simulink model "farmokinetic"  (R2015b)
settings: Solver=ode45  StartTime=0.0  StopTime=100  MaxStep=0.001  RelTol=1e-6
undefined symbols (not defined in the file): e, k1, k12, k21, kel, M, Time
libraries: dspswit3 x2
settings Model: Creator=DNikolaev  LastModifiedBy=DNikolaev

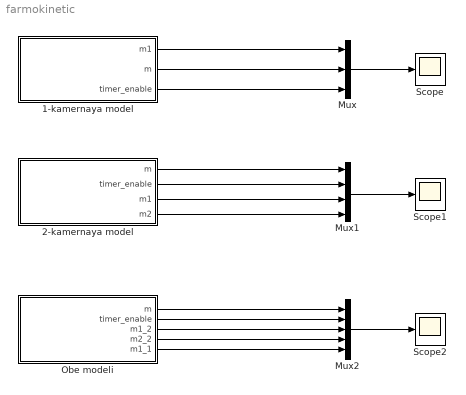
== system farmokinetic ==
  1-kamernaya model : Subsystem
  2-kamernaya model : Subsystem
  Mux : Mux  Inputs=3
  Mux1 : Mux
  Mux2 : Mux  Inputs=5
  Obe modeli : Subsystem
  Scope : Scope
  Scope1 : Scope
  Scope2 : Scope
  wires:
  1-kamernaya model/2(m) -> Mux/2
  1-kamernaya model/1(m1) -> Mux/1
  1-kamernaya model/3(timer_enable) -> Mux/3
  Mux/1 -> Scope/1
  2-kamernaya model/1(m) -> Mux1/1
  2-kamernaya model/2(timer_enable) -> Mux1/2
  Mux1/1 -> Scope1/1
  2-kamernaya model/3(m1) -> Mux1/3
  2-kamernaya model/4(m2) -> Mux1/4
  Mux2/1 -> Scope2/1
  Obe modeli/1(m) -> Mux2/1
  Obe modeli/2(timer_enable) -> Mux2/2
  Obe modeli/3(m1_2) -> Mux2/3
  Obe modeli/4(m2_2) -> Mux2/4
  Obe modeli/5(m1_1) -> Mux2/5

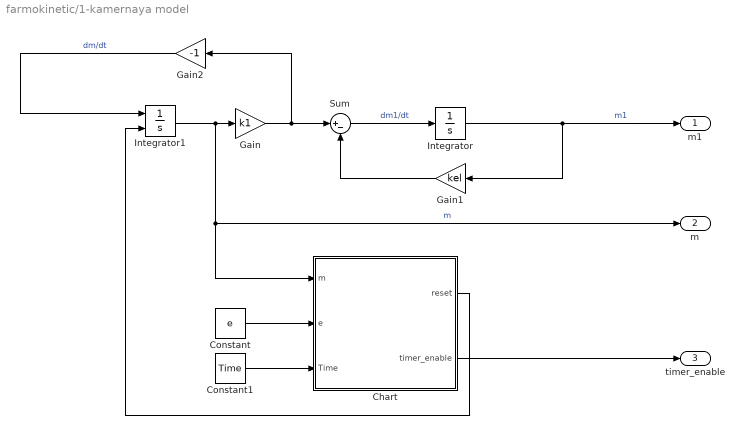
== system farmokinetic/1-kamernaya model ==
  Chart : Stateflow chart  TreatAsAtomicUnit=on
  Constant : Constant  Value=e
  Constant1 : Constant  Value=Time
  Gain : Gain  Gain=k1
  Gain1 : Gain  Gain=kel
  Gain2 : Gain  Gain=-1
  Integrator : Integrator
  Integrator1 : Integrator  ExternalReset=rising  InitialCondition=M
  Sum : Sum  Inputs=|+-
  m1 : Outport
  m : Outport  Port=2
  timer_enable : Outport  Port=3
  wires:
  Integrator/1 -> m1/1, Gain1/1  "m1"
  Sum/1 -> Integrator/1  "dm1/dt"
  Integrator1/1 -> Chart/1(m), m/1, Gain/1  "m"
  Gain/1 -> Gain2/1, Sum/1
  Gain1/1 -> Sum/2
  Gain2/1 -> Integrator1/1  "dm/dt"
  Chart/1(reset) -> Integrator1/2
  Chart/2(timer_enable) -> timer_enable/1
  Constant/1 -> Chart/2(e)
  Constant1/1 -> Chart/3(Time)

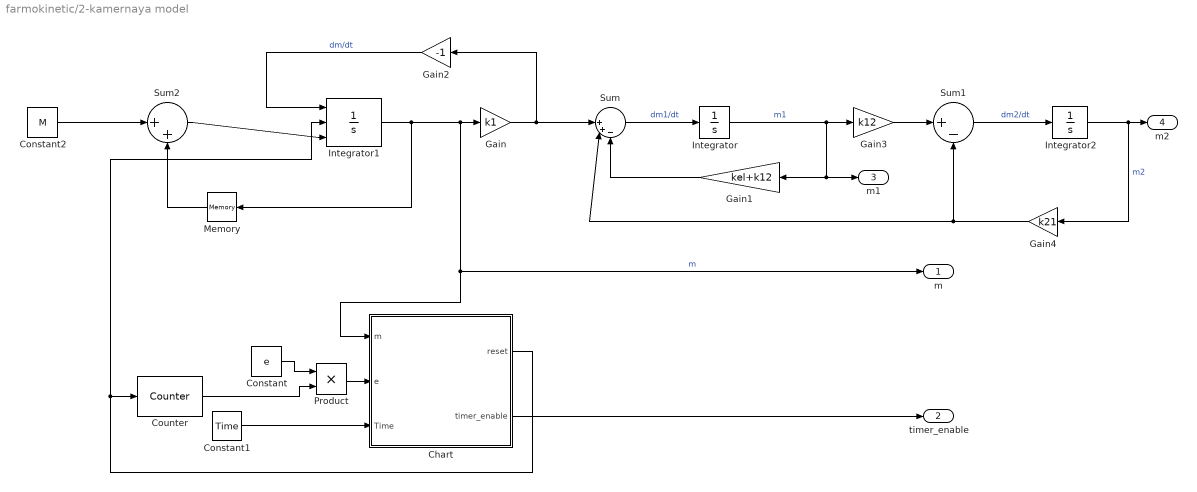
== system farmokinetic/2-kamernaya model ==
  Chart : Stateflow chart  TreatAsAtomicUnit=on
  Constant : Constant  Value=e
  Constant1 : Constant  Value=Time
  Constant2 : Constant  Value=M
  Counter : dspswit3/Counter  Direction=Up  CountEvent=Rising edge  CounterSize=User defined  MaxCount=50000  InitialCount=1  Output=Count  HitValue=32  ResetInput=off  SamplesPerFrame=1  Ts=1  CntDtype=double  HitDtype=Logical
  Gain : Gain  Gain=k1
  Gain1 : Gain  Gain=kel+k12
  Gain2 : Gain  Gain=-1
  Gain3 : Gain  Gain=k12
  Gain4 : Gain  Gain=k21
  Integrator : Integrator
  Integrator1 : Integrator  ExternalReset=rising  InitialConditionSource=external  InitialCondition=M
  Integrator2 : Integrator
  Memory : Memory
  Product : Product
  Sum : Sum  Inputs=||++-
  Sum1 : Sum  Inputs=|+-
  Sum2 : Sum  Inputs=|++
  m : Outport
  timer_enable : Outport  Port=2
  m1 : Outport  Port=3
  m2 : Outport  Port=4
  wires:
  Gain2/1 -> Integrator1/1  "dm/dt"
  Integrator1/1 -> Memory/1, Chart/1(m), m/1, Gain/1  "m"
  Gain1/1 -> Sum/3
  Gain/1 -> Sum/1, Gain2/1
  Sum/1 -> Integrator/1  "dm1/dt"
  Integrator/1 -> Gain1/1, m1/1, Gain3/1  "m1"
  Gain3/1 -> Sum1/1
  Integrator2/1 -> Gain4/1, m2/1  "m2"
  Gain4/1 -> Sum1/2, Sum/2
  Sum1/1 -> Integrator2/1  "dm2/dt"
  Constant2/1 -> Sum2/1
  Sum2/1 -> Integrator1/3
  Memory/1 -> Sum2/2
  Chart/1(reset) -> Integrator1/2, Counter/1
  Chart/2(timer_enable) -> timer_enable/1
  Constant/1 -> Product/1
  Constant1/1 -> Chart/3(Time)
  Product/1 -> Chart/2(e)
  Counter/1 -> Product/2

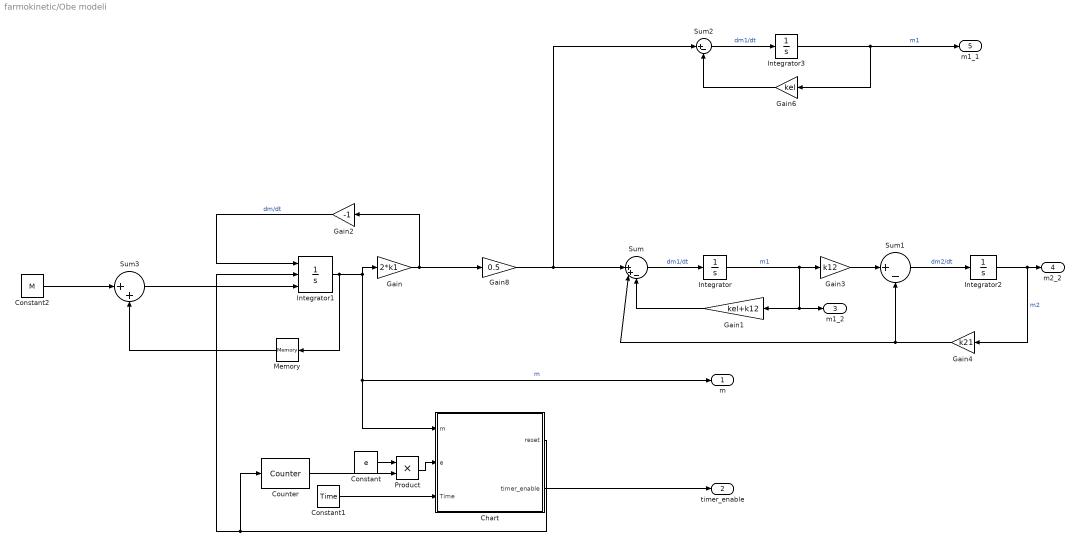
== system farmokinetic/Obe modeli ==
  Chart : Stateflow chart  TreatAsAtomicUnit=on
  Constant : Constant  Value=e
  Constant1 : Constant  Value=Time
  Constant2 : Constant  Value=M
  Counter : dspswit3/Counter  Direction=Up  CountEvent=Rising edge  CounterSize=User defined  MaxCount=50000  InitialCount=1  Output=Count  HitValue=32  ResetInput=off  SamplesPerFrame=1  Ts=1  CntDtype=double  HitDtype=Logical
  Gain : Gain  Gain=2*k1
  Gain1 : Gain  Gain=kel+k12
  Gain2 : Gain  Gain=-1
  Gain3 : Gain  Gain=k12
  Gain4 : Gain  Gain=k21
  Gain6 : Gain  Gain=kel
  Gain8 : Gain  Gain=0.5
  Integrator : Integrator
  Integrator1 : Integrator  ExternalReset=rising  InitialConditionSource=external  InitialCondition=M
  Integrator2 : Integrator
  Integrator3 : Integrator
  Memory : Memory
  Product : Product
  Sum : Sum  Inputs=||++-
  Sum1 : Sum  Inputs=|+-
  Sum2 : Sum  Inputs=|+-
  Sum3 : Sum  Inputs=|++
  m : Outport
  timer_enable : Outport  Port=2
  m1_2 : Outport  Port=3
  m2_2 : Outport  Port=4
  m1_1 : Outport  Port=5
  wires:
  Sum1/1 -> Integrator2/1  "dm2/dt"
  Gain4/1 -> Sum/2, Sum1/2
  Integrator2/1 -> m2_2/1, Gain4/1  "m2"
  Gain3/1 -> Sum1/1
  Integrator/1 -> Gain3/1, m1_2/1, Gain1/1  "m1"
  Sum/1 -> Integrator/1  "dm1/dt"
  Gain/1 -> Gain2/1, Gain8/1
  Gain1/1 -> Sum/3
  Integrator1/1 -> Memory/1, Gain/1, Chart/1(m), m/1  "m"
  Gain2/1 -> Integrator1/1  "dm/dt"
  Chart/1(reset) -> Counter/1, Integrator1/2
  Chart/2(timer_enable) -> timer_enable/1
  Constant/1 -> Product/1
  Constant1/1 -> Chart/3(Time)
  Integrator3/1 -> m1_1/1, Gain6/1  "m1"
  Sum2/1 -> Integrator3/1  "dm1/dt"
  Gain6/1 -> Sum2/2
  Gain8/1 -> Sum2/1, Sum/1
  Constant2/1 -> Sum3/1
  Sum3/1 -> Integrator1/3
  Memory/1 -> Sum3/2
  Product/1 -> Chart/2(e)
  Counter/1 -> Product/2

== stateflow chart farmokinetic/2-kamernaya model/Chart ==
  state Wait
    entry: reset=0;
    timer_enable=0;
  state Count
    entry: timer_enable=1;
  state Reset
    entry: reset=1;
  (default) -> Wait
  Reset -> Wait : after(0.1,sec)
  Count -> Wait [order 2] : [m>=e]
  Wait -> Count : [m<e]
  Count -> Reset [order 1] : after(Time,sec)
  data: m input; e input; Time input; reset output; timer_enable output

== stateflow chart farmokinetic/Obe modeli/Chart ==
  state Wait
    entry: reset=0;
    timer_enable=0;
  state Count
    entry: timer_enable=1;
  state Reset
    entry: reset=1;
  (default) -> Wait
  Reset -> Wait : after(0.1,sec)
  Count -> Wait [order 2] : [m>=e]
  Wait -> Count : [m<e]
  Count -> Reset [order 1] : after(Time,sec)
  data: m input; e input; Time input; reset output; timer_enable output

== stateflow chart farmokinetic/1-kamernaya model/Chart ==
  state Wait
    entry: reset=0;
    timer_enable=0;
  state Count
    entry: timer_enable=1;
  state Reset
    entry: reset=1;
  (default) -> Wait
  Reset -> Wait : after(0.1,sec)
  Count -> Wait [order 2] : [m>=e]
  Wait -> Count : [m<e]
  Count -> Reset [order 1] : after(Time,sec)
  data: m input; e input; Time input; reset output; timer_enable output
